simulink model "modelcomp"  (R2017a)
settings: Solver=VariableStepAuto  StartTime=0.0  StopTime=10  RelTol=1e-3
values from neighbouring files (symbols this model uses):
  R = r0*[1 -1]    [Param.m]
  S = [s1 s0]    [Param.m]
  Te = 1e-3    (= 0.001)    [Param.m]
settings Model: Creator=arek  LastModifiedBy=arek

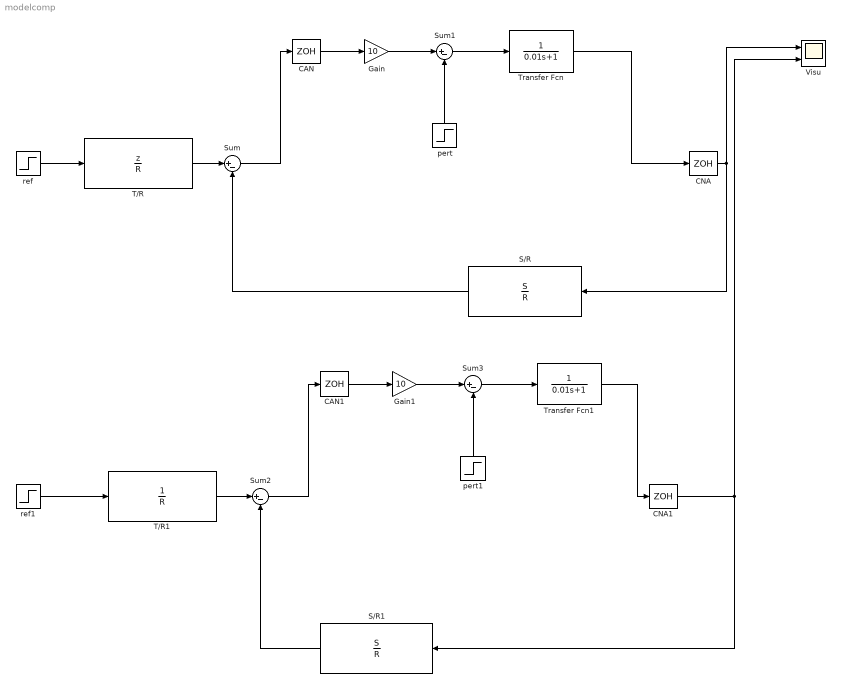
== system modelcomp ==
  CAN : ZeroOrderHold  SampleTime=-1
  CAN1 : ZeroOrderHold  SampleTime=-1
  CNA : ZeroOrderHold  SampleTime=-1
  CNA1 : ZeroOrderHold  SampleTime=-1
  Gain : Gain  Gain=10
  Gain1 : Gain  Gain=10
  S/R : DiscreteTransferFcn  Numerator=S  Denominator=R  SampleTime=Te
  S/R1 : DiscreteTransferFcn  Numerator=S  Denominator=R  SampleTime=Te
  Sum{,1..3} (4 alike) : Sum  Inputs=|+-
  T/R : DiscreteTransferFcn  Numerator=[1 0]  Denominator=R  SampleTime=Te
  T/R1 : DiscreteTransferFcn  Numerator=[0 1]  Denominator=R  SampleTime=Te
  Transfer Fcn : TransferFcn  Denominator=[0.01 1]
  Transfer Fcn1 : TransferFcn  Denominator=[0.01 1]
  Visu : Scope  NumInputPorts=2
  pert : Step  Time=5  SampleTime=Te
  pert1 : Step  Time=5  SampleTime=Te
  ref : Step  Time=0  SampleTime=Te
  ref1 : Step  Time=0  SampleTime=Te
  wires:
  S/R/1 -> Sum/2
  T/R/1 -> Sum/1
  Transfer Fcn/1 -> CNA/1
  CNA/1 -> S/R/1, Visu/1
  ref/1 -> T/R/1
  Sum/1 -> CAN/1
  CAN/1 -> Gain/1
  Gain/1 -> Sum1/1
  Sum1/1 -> Transfer Fcn/1
  pert/1 -> Sum1/2
  CAN1/1 -> Gain1/1
  Gain1/1 -> Sum3/1
  ref1/1 -> T/R1/1
  S/R1/1 -> Sum2/2
  Sum2/1 -> CAN1/1
  Transfer Fcn1/1 -> CNA1/1
  CNA1/1 -> Visu/2, S/R1/1
  pert1/1 -> Sum3/2
  T/R1/1 -> Sum2/1
  Sum3/1 -> Transfer Fcn1/1
